simulink model "variant_subsystem"  (R2018b)
settings: Solver=VariableStepAuto  StartTime=0.0  StopTime=10.0  RelTol=1e-3
settings Model: Creator=marwan  LastModifiedBy=marwan

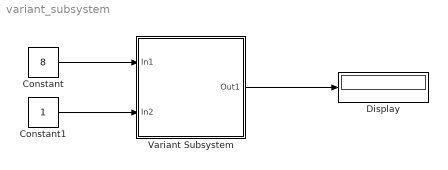
== system variant_subsystem ==
  Constant : Constant  Value=8
  Constant1 : Constant
  Display : Display
  Variant Subsystem : Subsystem  Variant=on
  wires:
  Variant Subsystem/1(Out1) -> Display/1
  Constant/1 -> Variant Subsystem/1(In1)
  Constant1/1 -> Variant Subsystem/2(In2)

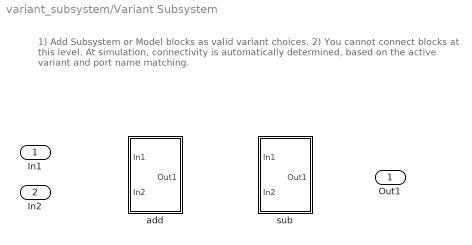
== system variant_subsystem/Variant Subsystem ==
  note: 1) Add Subsystem or Model blocks as valid variant choices.
      | 2) You cannot connect blocks at this level. At simulation, connectivity is automatically
      | determined, based on the active variant and port name matching.
  In1 : Inport
  In2 : Inport  Port=2
  add : Subsystem  VariantControl=addition
  sub : Subsystem  VariantControl=sub
  Out1 : Outport

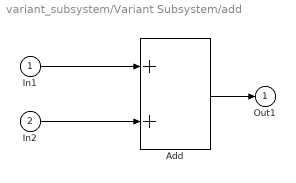
== system variant_subsystem/Variant Subsystem/add ==
  In1 : Inport
  In2 : Inport  Port=2
  Add : Sum
  Out1 : Outport
  wires:
  In1/1 -> Add/1
  Add/1 -> Out1/1
  In2/1 -> Add/2

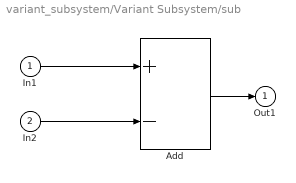
== system variant_subsystem/Variant Subsystem/sub ==
  In1 : Inport
  In2 : Inport  Port=2
  Add : Sum  Inputs=+-
  Out1 : Outport
  wires:
  In2/1 -> Add/2
  Add/1 -> Out1/1
  In1/1 -> Add/1
